simulink model "rtwdemo_rsim_param_tuning"  (Simulink 7.6)
settings: Solver=FixedStepDiscrete  StartTime=0.0  StopTime=48  FixedStep=1  RelTol=1e-3
PreLoadFcn:
  | clear;INC=uint8(1);LIMIT=uint8(16);K=int32(2);RESET=uint8(0);
StartFcn:
  | platform_finder('')
Description:
  | Interactive Parameter Tuning with RSim Target
settings Model: Creator=The MathWorks Inc.  CovMetricSettings=d  ExtModeTrigMode=oneshot  ExtModeArmWhenConnect=off  ExtModeAutoUpdateStatusClock=off  TunableVars=INC,LIMIT,RESET,K  TunableVarsStorageClass=ExportedGlobal,ExportedGlobal,ExportedGlobal,ExportedGlobal  TunableVarsTypeQualifier=,,,
settings MATStruct: SampleTime=1  Offset=0  Priority=[20.0]
settings DataIOCC: LimitDataPoints=off  SaveFormat=StructureWithTime  SignalLoggingName=sigsOut
settings OptimizationCC: InlineParams=on  InlineInvariantSignals=on  EfficientFloat2IntCast=on  EfficientMapNaN2IntZero=off  BufferReusableBoundary=off
settings DebuggingCC: SolverPrmCheckMsg=none  IntegerOverflowMsg=none  StrictBusMsg=ErrorOnBusTreatedAsVector
settings HardwareCC: ProdIntDivRoundTo=Zero  ProdEndianess=LittleEndian  ProdHWDeviceType=Generic->32-bit Embedded Processor  TargetHWDeviceType=Generic->32-bit Embedded Processor
settings RTWCC: SystemTargetFile=rsim.tlc  TLCOptions=-p0  TemplateMakefile=rsim_default_tmf  RTWVerbose=off  ProcessScript=rsim_make_rtw_hook
settings RSimTargetCC: TargetFcnLib=ansi_tfl_tmw.mat  TargetFunctionLibrary=ANSI_C  ERTMultiwordTypeDef=System defined  ERTCodeCoverageTool=None  ERTMultiwordLength=256  IsPILTarget=off  EnableShiftOperators=on  PortableWordSizes=off

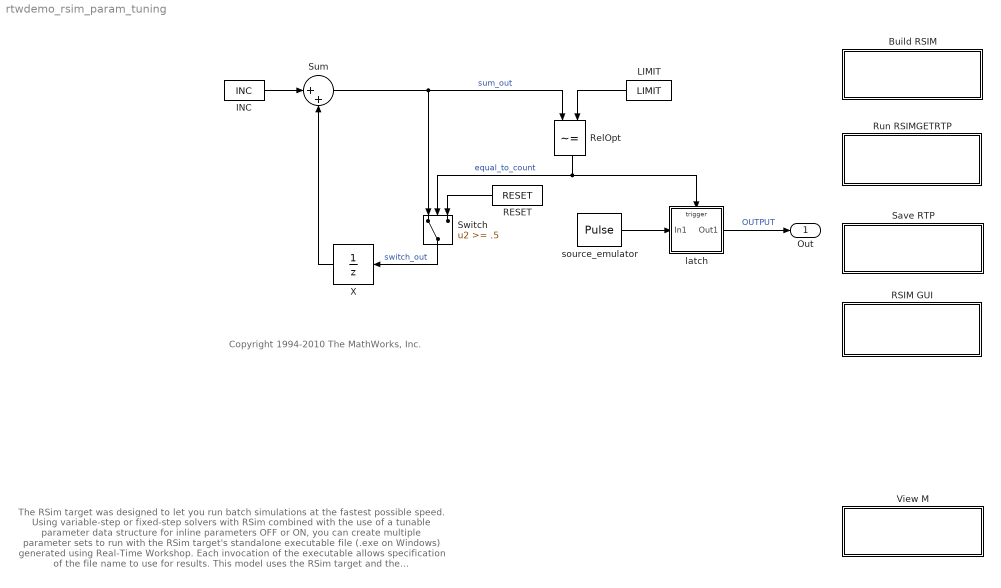
== system rtwdemo_rsim_param_tuning ==
  note: The RSim target was designed to let you run batch simulations at the fastest possible speed.
      | Using variable-step or fixed-step solvers with RSim combined with the use of a tunable
      | parameter data structure for inline parameters OFF or ON, you can create multiple parameter
      | sets to run with the RSim target's standalone executable file (.exe on Windows) generated
      | using Real-Time Workshop.  Each invocation of the executable allows specification of the file
      | name to use for results.
      |
      | This model uses the RSim target and the AddTunableParamInfo option in the RSIMGETRTP
      | function to allow a non-real-time executable to be passed new data without the need to
      | recompile the Simulink model. This feature allows you to easily get a map of the tunable
      | parameters declared in a model and save it in a MAT-file. You can then create your own
      | MATLAB GUI or a standalone GUI (independent of MATLAB) to read and write the MAT-file
      | and rerun the executable to produce new output files.
      |
      | Double-click the buttons at the upper right sequentially to run the demo.  To review the code
      | used to create both the MATLAB GUI and standalone GUI, double-click the View MATLAB programs button.
      |
      | For more information, you can also refer to the "Rapid Simulation Target" section in the
      | Real-Time Workshop documentation.
  note: Copyright 1994-2010 The MathWorks, Inc.
  Build RSIM : Subsystem
      settings: AttributesFormatString=\n\n\n\n\n\n\n\n
      settings: OpenFcn=|
      | platform_finder('')
      | disp('% ----- STEP 1: Building the Model with Real-Time Workshop ----- %')
      | rtwbuild('rtwdemo_rsim_param_tuning');
      mask Display: disp('1. Build Model with \n RSim Target')
  INC : Constant  Value=INC
  LIMIT : Constant  Value=LIMIT
  RESET : Constant  Value=RESET
  RSIM GUI : Subsystem
      settings: AttributesFormatString=\n\n\n\n\n\n\n\n
      settings: OpenFcn=|
      | disp(' ')
      | platform_finder('matlab_gui')
      mask Display: disp('4. Open the MATLAB \n RSIM GUI Demo')
  RelOpt : RelationalOperator  Operator=~=  InputSameDT=on
  Run RSIMGETRTP : Subsystem
      settings: AttributesFormatString=\n\n\n\n\n\n\n\n\n
      settings: OpenFcn=|
      | disp(' ')
      | disp('% ----- STEP 2 : Running the RSIMGETRTP command ----- %')
      | disp('>>rtp=rsimgetrtp(''rtwdemo_rsim_param_tuning'',''AddTunableParamInfo'',''on'')')
      | rtp=rsimgetrtp('rtwdemo_rsim_param_tuning','AddTunableParamInfo','on')
      | disp('% ----- Notice the ''map'' field of the structure ----- %')
      | disp('>>rtp.parameters')
      | rtp.parameters
      | disp('% ----- Here are the contents of the ''map'' field for the first parameter ----- %')
      | disp('>>rtp.parameters(1).map(1)')
      | rtp.parameters(1).map(1)
      mask Display: disp('2. Run RSIMGETRTP\nwith the option')
  Save RTP : Subsystem
      settings: AttributesFormatString=\n\n\n\n\n\n\n\n\n
      settings: OpenFcn=|
      | platform_finder('')
      | disp('% ----- STEP 3: Saving the rtp Structure in a MAT-File ----- %')
      | disp('>>save rsim_rtp_struct rtp')
      | save rsim_rtp_struct rtp
      mask Display: disp('3. Save RTP structure \n in a MAT-File')
  Sum : Sum  Inputs=|++  InputSameDT=on  OutDataTypeStr=Inherit: Same as first input
  Switch : Switch  Threshold=.5  InputSameDT=on
  View M : Subsystem
      settings: OpenFcn=edit('rsim_gui.m'); edit('rsim_gui_sa.m');
      mask Display: disp('View MATLAB programs')
  X : UnitDelay  StateIdentifier=X
      settings: RTWStateStorageClass=ExportedGlobal
  latch : Subsystem  TreatAsAtomicUnit=on
  source_emulator : DiscretePulseGenerator  Amplitude=int32(1)  Period=4  PulseWidth=2
  Out : Outport
  wires:
  INC/1 -> Sum/1
  X/1 -> Sum/2
  Switch/1 -> X/1  "switch_out"
  Sum/1 -> Switch/1, RelOpt/1  "sum_out"
  LIMIT/1 -> RelOpt/2
  RESET/1 -> Switch/3
  RelOpt/1 -> latch/Trigger, Switch/2  "equal_to_count"
  latch/1(Out1) -> Out/1  "OUTPUT"
  source_emulator/1 -> latch/1(In1)

== system rtwdemo_rsim_param_tuning/Build RSIM ==

== system rtwdemo_rsim_param_tuning/RSIM GUI ==

== system rtwdemo_rsim_param_tuning/Run RSIMGETRTP ==

== system rtwdemo_rsim_param_tuning/Save RTP ==

== system rtwdemo_rsim_param_tuning/View M ==

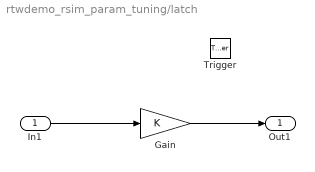
== system rtwdemo_rsim_param_tuning/latch ==
  In1 : Inport
  Trigger : TriggerPort  ZeroCross=off
  Gain : Gain  Gain=K  OutDataTypeStr=Inherit: Same as input  ParamDataTypeStr=Inherit: Same as input
  Out1 : Outport  InitialOutput=0
  wires:
  In1/1 -> Gain/1
  Gain/1 -> Out1/1
